simulink model "chap6_2sim"  (Simulink 7.7)
settings: Solver=ode45  StartTime=0.0  StopTime=10  RelTol=1e-3
settings Model: Creator=ljk  LastModifiedBy=ljk  ExtModeTrigMode=oneshot  ExtModeArmWhenConnect=off
settings DataIOCC: LimitDataPoints=off
settings OptimizationCC: BlockReduction=off  BooleanDataType=off
settings DebuggingCC: SaveWithParameterizedLinksMsg=none  SignalResolutionControl=TryResolveAllWithWarning  SolverPrmCheckMsg=none  MultiTaskDSMMsg=warning  MultiTaskCondExecSysMsg=none  StrictBusMsg=None
settings HardwareCC: TargetUnknown=on
settings RTWCC: IncludeERTFirstTime=on

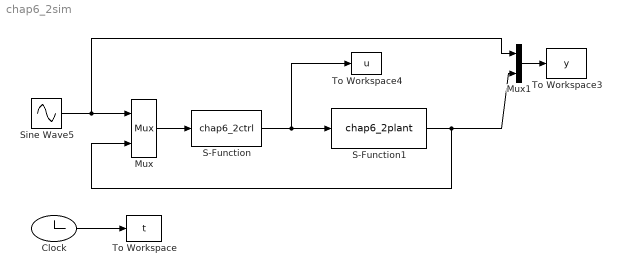
== system chap6_2sim ==
  Clock : Clock
  Mux : Mux  Inputs=2
  Mux1 : Mux  Inputs=2
  S-Function : S-Function  FunctionName=chap6_2ctrl  EnableBusSupport=off
  S-Function1 : S-Function  FunctionName=chap6_2plant  EnableBusSupport=off
  Sine Wave5 : Sin  SampleTime=0
  To Workspace : ToWorkspace  VariableName=t  SampleTime=-1  SaveFormat=Array
  To Workspace3 : ToWorkspace  VariableName=y  SampleTime=-1  SaveFormat=Array
  To Workspace4 : ToWorkspace  VariableName=u  SampleTime=-1  SaveFormat=Array
  wires:
  Mux/1 -> S-Function/1
  S-Function/1 -> S-Function1/1, To Workspace4/1
  S-Function1/1 -> Mux/2, Mux1/2
  Sine Wave5/1 -> Mux/1, Mux1/1
  Mux1/1 -> To Workspace3/1
  Clock/1 -> To Workspace/1
